simulink model "part_a"  (R2017b)
settings: Solver=VariableStepAuto  StartTime=0.0  StopTime=10.0  RelTol=1e-3
values from neighbouring files (symbols this model uses):
  a = [0 1;-1 -0.7]    [P2a.m]    (also in P2b.m; P2c.m)
  b = [0;1]    [P2a.m]    (also in P2b.m; P2c.m)
  c = [1 0;0 0]    [P2a.m]    (also in P2b.m; P2c.m = [1 0)
undefined symbols (not defined in the file or in its folder): K
settings Model: Creator=Soutrik  LastModifiedBy=Soutrik

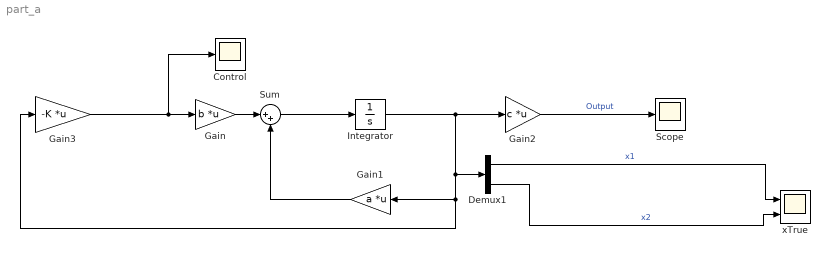
== system part_a ==
  Control : Scope
  Demux1 : Demux  Outputs=2
  Gain : Gain  Gain=b  Multiplication=Matrix(K*u)
  Gain1 : Gain  Gain=a  Multiplication=Matrix(K*u)
  Gain2 : Gain  Gain=c  Multiplication=Matrix(K*u)
  Gain3 : Gain  Gain=-K  Multiplication=Matrix(K*u)
  Integrator : Integrator  InitialCondition=[1 0]
  Scope : Scope
  Sum : Sum  Inputs=|++
  xTrue : Scope  NumInputPorts=2
  wires:
  Demux1/2 -> xTrue/2  "x2"
  Integrator/1 -> Gain3/1, Gain1/1, Demux1/1, Gain2/1
  Gain2/1 -> Scope/1  "Output"
  Demux1/1 -> xTrue/1  "x1"
  Gain3/1 -> Gain/1, Control/1
  Gain1/1 -> Sum/2
  Gain/1 -> Sum/1
  Sum/1 -> Integrator/1
